simulink model "SimLINbo"  (Simulink 7.0)
settings: Solver=ode45  StartTime=0.0  StopTime=10.0  RelTol=1e-3
values from neighbouring files (symbols this model uses):
  C = [1,0,0]    [DefParam.m]
undefined symbols (not defined in the file or in its folder): A, B
settings Model: Creator=Delphine  LastModifiedBy=Delphine

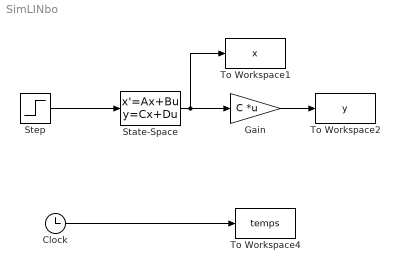
== system SimLINbo ==
  Clock : Clock
      settings: Decimation=10
  Gain : Gain  Gain=C  Multiplication=Matrix(K*u)  ParameterDataType=sfix(16)  ParameterScaling=2^0  OutDataType=sfix(16)  OutScaling=2^0
  State-Space : StateSpace  A=A  B=B  C=eye(3)  D=zeros(3,1)
  Step : Step  Time=2  After=0.3  SampleTime=0
  To Workspace1 : ToWorkspace  VariableName=x  SampleTime=-1  SaveFormat=Array
  To Workspace2 : ToWorkspace  VariableName=y  SampleTime=-1  SaveFormat=Array
  To Workspace4 : ToWorkspace  VariableName=temps  SampleTime=-1  SaveFormat=Array
  wires:
  Step/1 -> State-Space/1
  Clock/1 -> To Workspace4/1
  State-Space/1 -> Gain/1, To Workspace1/1
  Gain/1 -> To Workspace2/1
